simulink model "guidance_control_diagrams"  (Simulink 7.5)
settings: Solver=ode45  StartTime=0.0  StopTime=10.0  RelTol=1e-3
undefined symbols (not defined in the file): x, y, z
settings Model: Creator=tlmolloy  LastModifiedBy=tlmolloy
settings DebuggingCC: StrictBusMsg=Warning

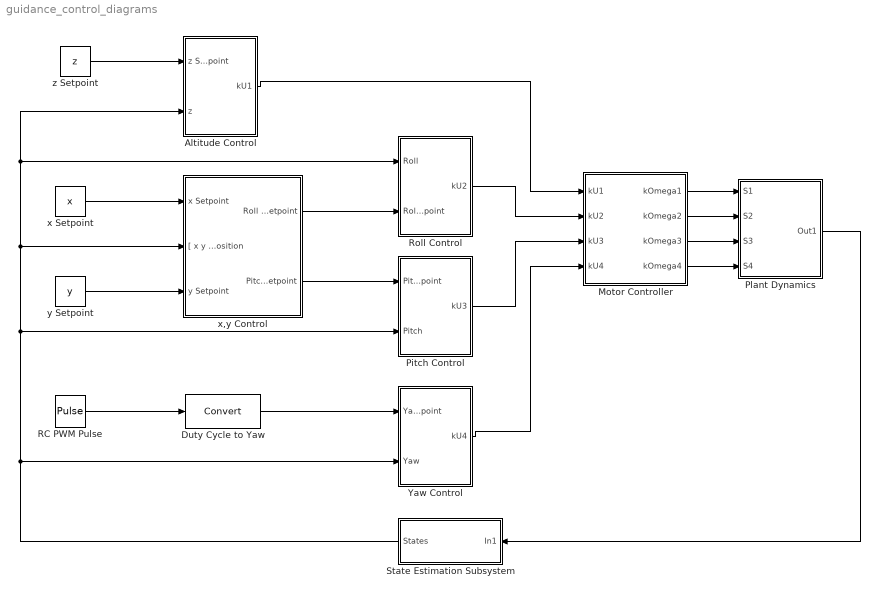
== system guidance_control_diagrams ==
  Altitude Control : Subsystem
  Duty Cycle to Yaw : DataTypeConversion  OutDataType=fixdt(1, 16)  OutScaling=2^0
  Motor Controller : Subsystem
  Pitch Control : Subsystem
  Plant Dynamics : Subsystem
  RC PWM Pulse : DiscretePulseGenerator  PulseType=Time based  Amplitude=1  Period=10  PulseWidth=5  PhaseDelay=0  SampleTime=1
  Roll Control : Subsystem
  State Estimation Subsystem : Subsystem
  Yaw Control : Subsystem
  x Setpoint : Constant  Value=x  OutDataType=fixdt(1, 16)  OutScaling=2^0
  x,y Control : Subsystem
  y Setpoint : Constant  Value=y  OutDataType=fixdt(1, 16)  OutScaling=2^0
  z Setpoint : Constant  Value=z  OutDataType=fixdt(1, 16)  OutScaling=2^0
  wires:
  Plant Dynamics/1(Out1) -> State Estimation Subsystem/1(In1)
  Motor Controller/1(kOmega1) -> Plant Dynamics/1(S1)
  Motor Controller/2(kOmega2) -> Plant Dynamics/2(S2)
  Motor Controller/3(kOmega3) -> Plant Dynamics/3(S3)
  Motor Controller/4(kOmega4) -> Plant Dynamics/4(S4)
  State Estimation Subsystem/1(States) -> x,y Control/2("[ x y ] Position"), Altitude Control/2(z), Roll Control/1(Roll), Pitch Control/2(Pitch), Yaw Control/2(Yaw)
  Altitude Control/1(kU1) -> Motor Controller/1(kU1)
  z Setpoint/1 -> Altitude Control/1(z Setpoint)
  x Setpoint/1 -> x,y Control/1(x Setpoint)
  y Setpoint/1 -> x,y Control/3(y Setpoint)
  x,y Control/1(Roll Setpoint) -> Roll Control/2(Roll Setpoint)
  Roll Control/1(kU2) -> Motor Controller/2(kU2)
  Pitch Control/1(kU3) -> Motor Controller/3(kU3)
  x,y Control/2(Pitch Setpoint) -> Pitch Control/1(Pitch Setpoint)
  Yaw Control/1(kU4) -> Motor Controller/4(kU4)
  RC PWM Pulse/1 -> Duty Cycle to Yaw/1
  Duty Cycle to Yaw/1 -> Yaw Control/1(Yaw Setpoint)

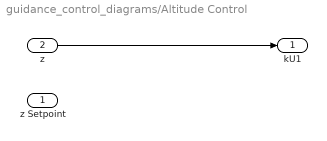
== system guidance_control_diagrams/Altitude Control ==
  z Setpoint : Inport  OutDataType=fixdt(1, 16)  OutScaling=2^0
  z : Inport  Port=2  OutDataType=fixdt(1, 16)  OutScaling=2^0
  kU1 : Outport  OutDataType=fixdt(1, 16)  OutScaling=2^0
  wires:
  z/1 -> kU1/1

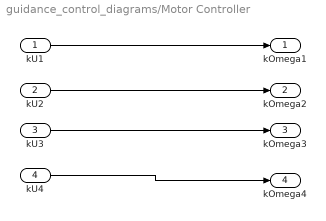
== system guidance_control_diagrams/Motor Controller ==
  kU1 : Inport  OutDataType=fixdt(1, 16)  OutScaling=2^0
  kU2 : Inport  Port=2  OutDataType=fixdt(1, 16)  OutScaling=2^0
  kU3 : Inport  Port=3  OutDataType=fixdt(1, 16)  OutScaling=2^0
  kU4 : Inport  Port=4  OutDataType=fixdt(1, 16)  OutScaling=2^0
  kOmega1 : Outport  OutDataType=fixdt(1, 16)  OutScaling=2^0
  kOmega2 : Outport  Port=2  OutDataType=fixdt(1, 16)  OutScaling=2^0
  kOmega3 : Outport  Port=3  OutDataType=fixdt(1, 16)  OutScaling=2^0
  kOmega4 : Outport  Port=4  OutDataType=fixdt(1, 16)  OutScaling=2^0
  wires:
  kU1/1 -> kOmega1/1
  kU2/1 -> kOmega2/1
  kU3/1 -> kOmega3/1
  kU4/1 -> kOmega4/1

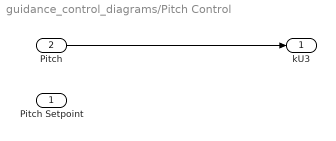
== system guidance_control_diagrams/Pitch Control ==
  Pitch Setpoint : Inport  OutDataType=fixdt(1, 16)  OutScaling=2^0
  Pitch : Inport  Port=2  OutDataType=fixdt(1, 16)  OutScaling=2^0
  kU3 : Outport  OutDataType=fixdt(1, 16)  OutScaling=2^0
  wires:
  Pitch/1 -> kU3/1

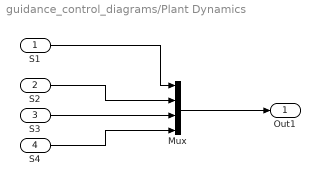
== system guidance_control_diagrams/Plant Dynamics ==
  S1 : Inport  OutDataType=fixdt(1, 16)  OutScaling=2^0
  S2 : Inport  Port=2  OutDataType=fixdt(1, 16)  OutScaling=2^0
  S3 : Inport  Port=3  OutDataType=fixdt(1, 16)  OutScaling=2^0
  S4 : Inport  Port=4  OutDataType=fixdt(1, 16)  OutScaling=2^0
  Mux : Mux
  Out1 : Outport  OutDataType=fixdt(1, 16)  OutScaling=2^0
  wires:
  S2/1 -> Mux/2
  S3/1 -> Mux/3
  S4/1 -> Mux/4
  S1/1 -> Mux/1
  Mux/1 -> Out1/1

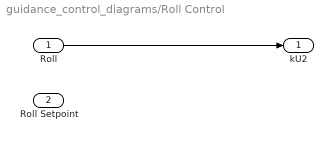
== system guidance_control_diagrams/Roll Control ==
  Roll : Inport  OutDataType=fixdt(1, 16)  OutScaling=2^0
  Roll Setpoint : Inport  Port=2  OutDataType=fixdt(1, 16)  OutScaling=2^0
  kU2 : Outport  OutDataType=fixdt(1, 16)  OutScaling=2^0
  wires:
  Roll/1 -> kU2/1

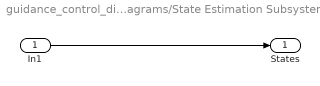
== system guidance_control_diagrams/State Estimation Subsystem ==
  In1 : Inport  OutDataType=fixdt(1, 16)  OutScaling=2^0
  States : Outport  OutDataType=fixdt(1, 16)  OutScaling=2^0
  wires:
  In1/1 -> States/1

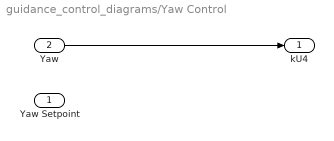
== system guidance_control_diagrams/Yaw Control ==
  Yaw Setpoint : Inport  OutDataType=fixdt(1, 16)  OutScaling=2^0
  Yaw : Inport  Port=2  OutDataType=fixdt(1, 16)  OutScaling=2^0
  kU4 : Outport  OutDataType=fixdt(1, 16)  OutScaling=2^0
  wires:
  Yaw/1 -> kU4/1

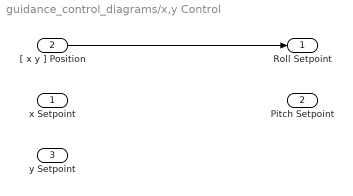
== system guidance_control_diagrams/x,y Control ==
  x Setpoint : Inport  OutDataType=fixdt(1, 16)  OutScaling=2^0
  "[ x y ] Position" : Inport  Port=2  OutDataType=fixdt(1, 16)  OutScaling=2^0
  y Setpoint : Inport  Port=3  OutDataType=fixdt(1, 16)  OutScaling=2^0
  Roll Setpoint : Outport  OutDataType=fixdt(1, 16)  OutScaling=2^0
  Pitch Setpoint : Outport  Port=2  OutDataType=fixdt(1, 16)  OutScaling=2^0
  wires:
  "[ x y ] Position"/1 -> Roll Setpoint/1
